simulink model "Lidar_Slam_Sim"  (R2022a)
settings: Solver=FixedStepAuto  StartTime=0.0  StopTime=inf  RelTol=1e-3
model workspace (MAT data in the model file):
  SL_ROS_VariableLengthArrays_MaxSizes.CommonInfo.ArrayTruncateAction = 'EmitWarning'
  SL_ROS_VariableLengthArrays_MaxSizes.MsgTypeMap = containers.Map
  SL_ROS_VariableLengthArrays_MaxSizes.MsgTypeMap.serialization.keys = {'sensor_msgs/LaserScan'}
  SL_ROS_VariableLengthArrays_MaxSizes.MsgTypeMap.serialization.values{1}(1).PropertyName = 'Intensities'
  SL_ROS_VariableLengthArrays_MaxSizes.MsgTypeMap.serialization.values{1}(1).DataType = 'single'
  SL_ROS_VariableLengthArrays_MaxSizes.MsgTypeMap.serialization.values{1}(1).MaxLength = 1081
  SL_ROS_VariableLengthArrays_MaxSizes.MsgTypeMap.serialization.values{1}(2).PropertyName = 'Ranges'
  SL_ROS_VariableLengthArrays_MaxSizes.MsgTypeMap.serialization.values{1}(2).DataType = 'single'
  SL_ROS_VariableLengthArrays_MaxSizes.MsgTypeMap.serialization.values{1}(2).MaxLength = 1081
  SL_ROS_VariableLengthArrays_MaxSizes.MsgTypeMap.serialization.uniformity = 0
  SL_ROS_VariableLengthArrays_MaxSizes.MsgTypeMap.serialization.keyType = 'char'
  SL_ROS_VariableLengthArrays_MaxSizes.MsgTypeMap.serialization.valueType = 'any'
values from neighbouring files (symbols this model uses):
  pose = poses(end,:)    [LidarSlam.m]    (also in LidarSlam_interp.m)
  scan = lidarScan(ranges,angles)    [LidarSlam.m]    (also in LidarSlam_interp.m)
  slamStatus = int8(1)    [LidarSlam.m]    (also in LidarSlam_interp.m)
undefined symbols (not defined in the file or in its folder): Angular, Linear, Theta, X, Y
libraries: robotlib x7, visionsinks x1
settings Model: Creator=Ron  LastModifiedBy=josea
settings OptimizationCC: EnhancedBackFolding=on  PassReuseOutputArgsAs=Individual arguments  ZeroExternalMemoryAtStartup=off  ZeroInternalMemoryAtStartup=off  MaxStackSize=64  OptimizeBlockOrder=speed  DifferentSizesBufferReuse=on  OptimizationCustomize=off  EfficientTunableParamExpr=on
settings DebuggingCC: ParameterTunabilityLossMsg=error  UnconnectedInputMsg=warning  UnconnectedOutputMsg=warning  UnconnectedLineMsg=warning
settings HardwareCC: ProdBitPerPointer=32  ProdBitPerSizeT=32  ProdBitPerPtrDiffT=32  ProdLargestAtomicFloat=None  ProdIntDivRoundTo=Undefined  ProdEndianess=Unspecified  ProdWordSize=32  ProdHWDeviceType=Generic->Unspecified (assume 32-bit Generic)
settings RTWCC: SystemTargetFile=ert.tlc  HardwareBoard=Robot Operating System (ROS)  TLCOptions="-aInlineSetEventsForThisBaseRateFcn=TLC_FALSE -aSuppressMultiTaskScheduler=TLC_FALSE    -aRateBasedStepFcn=0"  TemplateMakefile=ert_default_tmf  Toolchain=Catkin  TargetLang=C++  DLArmComputeVersion=19.05
settings CodeAppCC: ForceParamTrailComments=on  IgnoreCustomStorageClasses=off  OperatorAnnotations=on  SimulinkDataObjDesc=on  SFDataObjDesc=on  InsertBlockDesc=on
settings ERTTargetCC: SupportVariableSizeSignals=on  ExtModeMexArgs='192.168.80.136' 0 17725  RootIOFormat=Structure reference

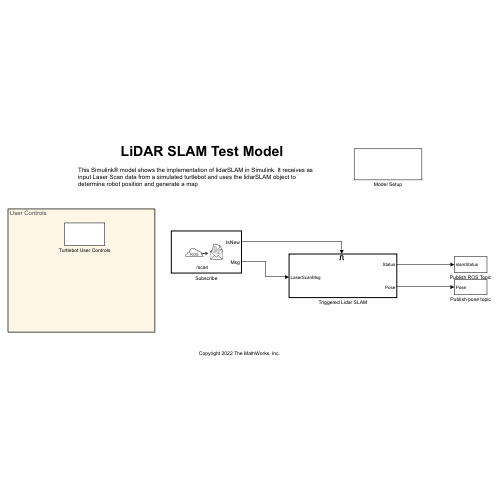
[thumbnail: Simulink's stored preview of the top-level diagram]
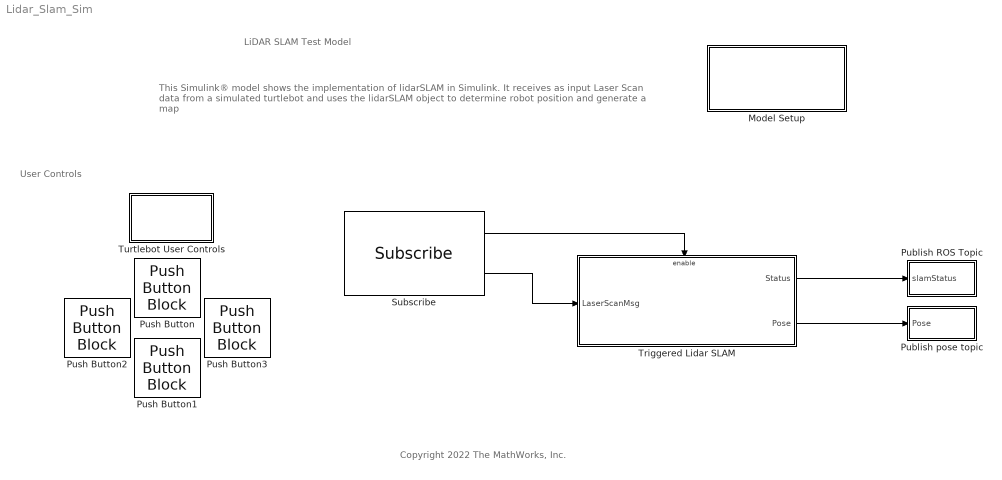
== system Lidar_Slam_Sim ==
  note: LiDAR SLAM Test Model
  note: This Simulink® model shows the implementation of lidarSLAM in Simulink. It receives as input Laser Scan data from a simulated turtlebot and uses the lidarSLAM object to determine robot position and generate a map
  note: Copyright 2022 The MathWorks, Inc.
  note: User Controls
  Model Setup : Subsystem
  Publish ROS Topic : Subsystem
  Publish pose topic : Subsystem
  Push Button : PushButtonBlock  ButtonText=Fwd  OffValue=0.000000
  Push Button1 : PushButtonBlock  ButtonText=Rev  OnValue=-1  OffValue=0.000000
  Push Button2 : PushButtonBlock  ButtonText=Left  OffValue=0.000000
  Push Button3 : PushButtonBlock  ButtonText=Right  OnValue=-1  OffValue=0.000000
  Subscribe : robotlib/Subscribe  topicSource=Select from ROS network  topic=/scan  messageType=sensor_msgs/LaserScan  SampleTime=0.5  legacyBusStruct=off  messageQueueLength=1
  Triggered Lidar SLAM : Subsystem
  Turtlebot User Controls : Subsystem
  wires:
  Subscribe/1 -> Triggered Lidar SLAM/Enable
  Subscribe/2 -> Triggered Lidar SLAM/1(LaserScanMsg)
  Triggered Lidar SLAM/1(Status) -> Publish ROS Topic/1(slamStatus)
  Triggered Lidar SLAM/2(Pose) -> Publish pose topic/1(Pose)

== system Lidar_Slam_Sim/Model Setup ==
  note: Before running the Simulink model, make sure the ROS network requirements have been set appropriately through the Simulink Toolstrip. Note that setting a Node Host IP address is optional and depends on the computer setup.
  note: ROS Model Setup

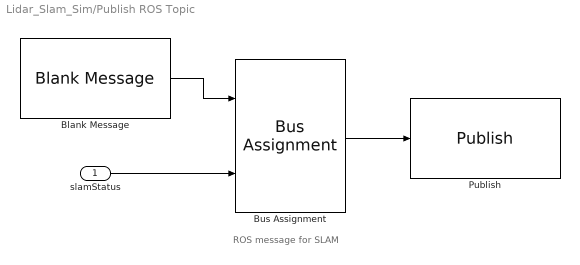
== system Lidar_Slam_Sim/Publish ROS Topic ==
  note: ROS message for SLAM
  slamStatus : Inport
  Blank Message : robotlib/Blank Message  messageClass=Message  entityType=std_msgs/Int8  messageType=std_msgs/Int8  SampleTime=inf  legacyBusStruct=off
  Bus Assignment : BusAssignment  AssignedSignals=Data
  Publish : robotlib/Publish  topicSource=Specify your own  topic=/slamStatus  messageType=std_msgs/Int8  legacyBusStruct=off  messageQueueLength=1
  wires:
  Bus Assignment/1 -> Publish/1
  Blank Message/1 -> Bus Assignment/1
  slamStatus/1 -> Bus Assignment/2

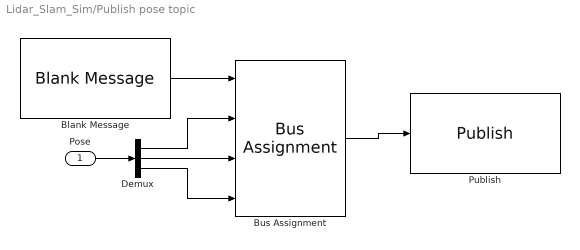
== system Lidar_Slam_Sim/Publish pose topic ==
  Pose : Inport
  Blank Message : robotlib/Blank Message  messageClass=Message  entityType=geometry_msgs/Pose2D  messageType=geometry_msgs/Pose2D  SampleTime=inf  legacyBusStruct=off
  Bus Assignment : BusAssignment  AssignedSignals=X,Y,Theta
  Demux : Demux  Outputs=3
  Publish : robotlib/Publish  topicSource=Specify your own  topic=/pose  messageType=geometry_msgs/Pose2D  legacyBusStruct=off  messageQueueLength=1
  wires:
  Blank Message/1 -> Bus Assignment/1
  Bus Assignment/1 -> Publish/1
  Pose/1 -> Demux/1
  Demux/3 -> Bus Assignment/4
  Demux/1 -> Bus Assignment/2
  Demux/2 -> Bus Assignment/3

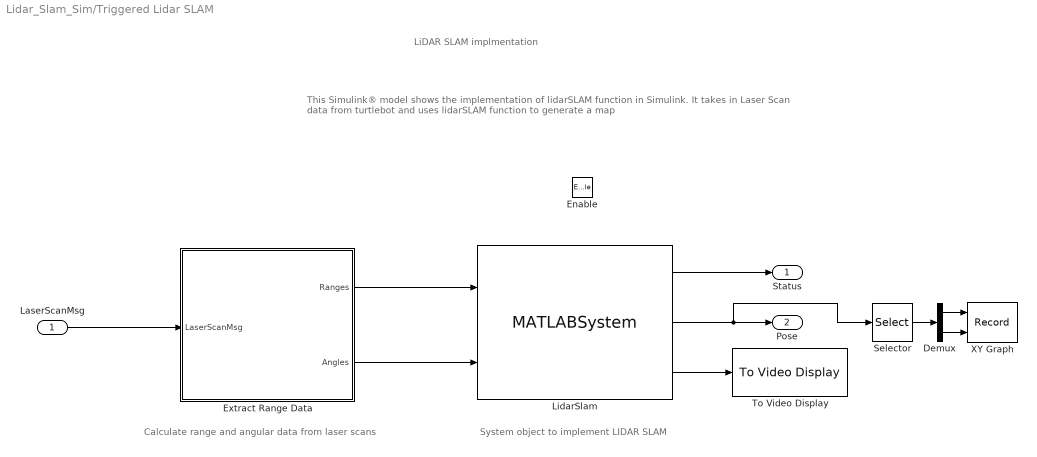
== system Lidar_Slam_Sim/Triggered Lidar SLAM ==
  note: Calculate range and angular data from laser scans
  note: LiDAR SLAM implmentation
  note: This Simulink® model shows the implementation of lidarSLAM function in Simulink. It takes in Laser Scan data from turtlebot and uses lidarSLAM function to generate a map
  note: System object to implement LIDAR SLAM
  LaserScanMsg : Inport
  Enable : EnablePort  PropagateVarSize=During execution
  Demux : Demux  Outputs=2
  Extract Range Data : MATLAB Function  TreatAsAtomicUnit=on
  LidarSlam : MATLABSystem  System=LidarSlam_interp  SimulateUsing=Interpreted execution
      mask Type: LidarSlam_interp
      mask Display:
      | disp('LidarSlam_interp');
      | port_label('input',1,'ranges');
      | port_label('input',2,'angles');
      | port_label('output',1,'slamStatus');
      | port_label('output',2,'pose');
      | port_label('output',3,'mapData');
  Selector : Selector  InputPortWidth=3  IndexOptions=Index vector (dialog)  Indices=[1 2]  OutputSizes=1
  To Video Display : visionsinks/To Video Display  windowSizeMode=Normal  openAtMdlStart=on  fullScreen=off  videoWindowX=2818  videoWindowY=107  saveWindowSize=off  videoWindowWidth=1000  videoWindowHeight=1000  inputColorFormat=RGB  inputType=Obsolete  imagePorts=One multidimensional signal  OutputDevice=On-screen video monitor  dataOrg=Column-major  isWindowOpen=off
  XY Graph : Record  FileSettingsInternal="{\"entries\":[{\"content\":{\"excelSettings\":{\"content\":{},\"type\":\"Streamout.ExcelSettings\"}},\"type\":\"Streamout.FileSettingStorage\",\"uuid\":\"e6529120-ae98-45b0-a233-f6222d18b903\"}],\"packageUris\":[\"http://schema.mathworks.com/mf0/streamout_blocks/R2020a\"],\"version\":\"1.0\"}"  Layout=[1 1]  SignalsInternal="{\"entries\":[{\"content\":{\"signals\":[{\"content\":{\"blockPath\":[\"Lidar_Slam_Test_22a/Triggered Lidar SLAM/XY Graph\"],\"channel\":[],\"dimensions\":[1,1],\"domain\":\"Lidar_Slam_Test_22a/Triggered Lidar SLAM/XY Graph\",\"lineColor\":\"#a2142f\",\"plots\":[1],\"port\":1,\"sid\":[],\"signalID\":659,\"signalName\":\"Demux:1\"},\"type\":\"RecordBlkView.Signal\",\"uuid\":\"5e7170b5-bad1-49cf-a93f-00d98687c61b\"},{\"content\":{\"blockPath\":[\"Lidar_Slam_Test_22a/Triggered Lidar SLAM/XY Graph\"],\"channel\":[],\"dimensions\":[1,1],\"domain\":\"Lidar_Slam_Test_22a/Triggered Lidar SLAM/XY Graph\",\"lineColor\":\"#139fff\",\"plots\":[1],\"port\":2,\"sid\":[],\"signalID\":662,\"signalName\":\"Demux:2\"},\"type\":\"RecordBlkView.Signal\",\"uuid\":\"e2b85a74-b7ed-4e83-89e4-ad117cd42b8d\"}]},\"type\":\"RecordBlkView.InputSignals\",\"uuid\":\"800c35c5-dc7b-43f4-bb38-1d32d61184ba\"}],\"packageUris\":[\"http://schema.mathworks.com/mf0/streamout_blocks/R2020a\"],\"version\":\"1.0\"}"  VisualizationBindings="{\"xyplotplugin\":{\"info\":[{\"series\":[{\"bindingParametersList\":[{\"parameter\":\"X-Axis\",\"signalID\":659,\"signalName\":\"Demux:1\"},{\"parameter\":\"Y-Axis\",\"signalID\":662,\"signalName\":\"Demux:2\"}],\"seriesID\":9056}],\"subplotID\":1}]}}"  CompatibilityTag=XY  st=-1
  Status : Outport
  Pose : Outport  Port=2
  wires:
  LaserScanMsg/1 -> Extract Range Data/1(LaserScanMsg)
  Extract Range Data/1(Ranges) -> LidarSlam/1
  Extract Range Data/2(Angles) -> LidarSlam/2
  LidarSlam/1 -> Status/1
  LidarSlam/2 -> Pose/1, Selector/1
  Demux/2 -> XY Graph/2
  Demux/1 -> XY Graph/1
  Selector/1 -> Demux/1
  LidarSlam/3 -> To Video Display/1

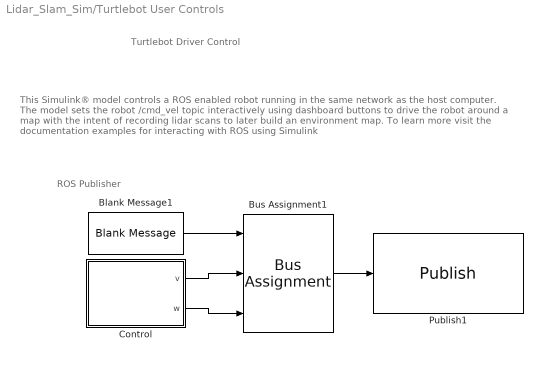
== system Lidar_Slam_Sim/Turtlebot User Controls ==
  note: Turtlebot Driver Control
  note: ROS Publisher
  note: This Simulink® model controls a ROS enabled robot running in the same network as the host computer. The model sets the robot /cmd_vel topic interactively using dashboard buttons to drive the robot around a map with the intent of recording lidar scans to later build an environment map. To learn more visit the documentation examples for interacting with ROS using Simulink
  Blank Message1 : robotlib/Blank Message  messageClass=Message  entityType=geometry_msgs/Twist  messageType=geometry_msgs/Twist  SampleTime=0.1  legacyBusStruct=off
  Bus Assignment1 : BusAssignment  AssignedSignals=Linear.X,Angular.Z
  Control : Subsystem
  Publish1 : robotlib/Publish  topicSource=Select from ROS network  topic=/cmd_vel  messageType=geometry_msgs/Twist  legacyBusStruct=off  messageQueueLength=1
  wires:
  Control/2(w) -> Bus Assignment1/3
  Control/1(v) -> Bus Assignment1/2
  Blank Message1/1 -> Bus Assignment1/1
  Bus Assignment1/1 -> Publish1/1

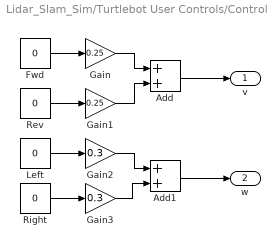
== system Lidar_Slam_Sim/Turtlebot User Controls/Control ==
  Add : Sum
  Add1 : Sum
  Fwd : Constant  Value=0
  Gain : Gain  Gain=0.25
  Gain1 : Gain  Gain=0.25
  Gain2 : Gain  Gain=0.3
  Gain3 : Gain  Gain=0.3
  Left : Constant  Value=0
  Rev : Constant  Value=0
  Right : Constant  Value=0
  v : Outport
  w : Outport  Port=2
  wires:
  Rev/1 -> Gain1/1
  Add/1 -> v/1
  Left/1 -> Gain2/1
  Fwd/1 -> Gain/1
  Right/1 -> Gain3/1
  Add1/1 -> w/1
  Gain/1 -> Add/1
  Gain1/1 -> Add/2
  Gain2/1 -> Add1/1
  Gain3/1 -> Add1/2

== matlab function Lidar_Slam_Sim/Triggered Lidar SLAM/Extract Range Data ==
  data: LaserScanMsg input; Ranges output; Angles output
function [Ranges, Angles] = ExtractRangeData(LaserScanMsg)
%#codegen

% Extract Range information
Ranges = double(LaserScanMsg.Ranges);

% Construct Angles vector using AngleMin and AngleIncrement from sensor
% reading.
angMin = double(LaserScanMsg.AngleMin);
angIncrement = double(LaserScanMsg.AngleIncrement);

numReadings = numel(Ranges);
rawAngles = angMin + (0:numReadings-1)' * angIncrement;

% Wrap the angles to the (-pi,pi] interval.
Angles = robotics.internal.wrapToPi(double(rawAngles));
